simulink model "qpsk_rx_ssr_hb_decim"  (R2020a)
settings: Solver=VariableStepAuto  StartTime=0.0  StopTime=10000/64e6  RelTol=1e-3
PreLoadFcn:
  | setup_qpsk_receiver
InitFcn:
  | setup_qpsk_receiver
values from neighbouring files (symbols this model uses):
  tx_data = [tx_data mbuf]    [setup_receiver.m]
undefined symbols (not defined in the file or in its folder): designMultirateFIR, xlfda_numerator
libraries: xbsIndex_r4 x13, hdlsllib x9, dspmlti4 x8, xrbsSSR_Library x4, dspswit3 x4, commrandsrc3 x2, dspsigops x2, simulink x1
(part 1 of 2)
settings Model: Creator=david  LastModifiedBy=david
settings SFSimCC: CustomCodeUndefinedFunction=UseInterfaceOnly

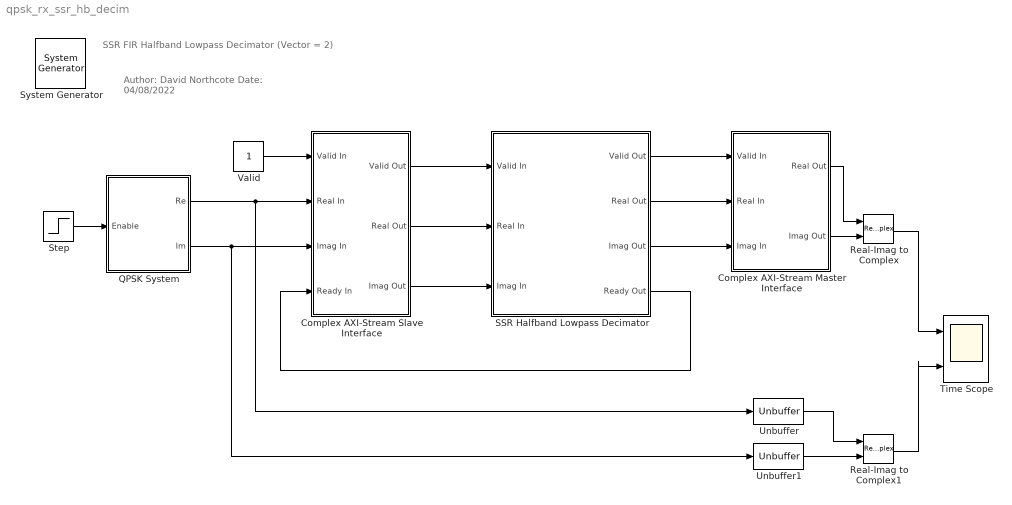
== system qpsk_rx_ssr_hb_decim ==
  note: Author: 	David Northcote
      | Date: 	04/08/2022
  note: SSR FIR Halfband Lowpass Decimator (Vector = 2)
  " System Generator" : xbsIndex_r4/ System Generator  Tag=genX  xilinxfamily=zynquplusRFSOC  part=xczu28dr  speed=-2-e  package=ffvg1517  synthesis_tool=Vivado  clock_wrapper=Clock Enables  directory=./netlist  proj_type=Vivado  Synth_file=Vivado Synthesis Defaults  Impl_file=Vivado Implementation Defaults  testbench=off  simulink_period=1/64e6  sysclk_period=(1/64e6)*1e9  dcm_input_clock_period=10  incr_netlist=off  trim_vbits=Everywhere in SubSystem  dbl_ovrd=According to Block Masks  core_generation=According to Block Masks  run_coregen=off  deprecated_control=off  eval_field=0  block_type=sysgen
  Complex AXI-Stream Master Interface : Subsystem
  Complex AXI-Stream Slave Interface : Subsystem
  QPSK System : Subsystem
  Real-Imag to Complex : RealImagToComplex
  Real-Imag to Complex1 : RealImagToComplex
  SSR Halfband Lowpass Decimator : Subsystem
  Step : Step  Time=2/25e3  SampleTime=1/25e3
  Time Scope : Scope  NumInputPorts=2
  Unbuffer : Unbuffer
  Unbuffer1 : Unbuffer
  Valid : Constant  OutDataTypeStr=boolean  SampleTime=1/64e6
  wires:
  QPSK System/1(Re) -> Unbuffer/1, Complex AXI-Stream Slave Interface/2(Real In)
  QPSK System/2(Im) -> Unbuffer1/1, Complex AXI-Stream Slave Interface/3(Imag In)
  Step/1 -> QPSK System/1(Enable)
  Unbuffer1/1 -> Real-Imag to Complex1/2
  Unbuffer/1 -> Real-Imag to Complex1/1
  Real-Imag to Complex1/1 -> Time Scope/2
  Real-Imag to Complex/1 -> Time Scope/1
  SSR Halfband Lowpass Decimator/1(Valid Out) -> Complex AXI-Stream Master Interface/1(Valid In)
  SSR Halfband Lowpass Decimator/2(Real Out) -> Complex AXI-Stream Master Interface/2(Real In)
  SSR Halfband Lowpass Decimator/3(Imag Out) -> Complex AXI-Stream Master Interface/3(Imag In)
  Complex AXI-Stream Master Interface/1(Real Out) -> Real-Imag to Complex/1
  Complex AXI-Stream Master Interface/2(Imag Out) -> Real-Imag to Complex/2
  Valid/1 -> Complex AXI-Stream Slave Interface/1(Valid In)
  SSR Halfband Lowpass Decimator/4(Ready Out) -> Complex AXI-Stream Slave Interface/4(Ready In)
  Complex AXI-Stream Slave Interface/1(Valid Out) -> SSR Halfband Lowpass Decimator/1(Valid In)
  Complex AXI-Stream Slave Interface/2(Real Out) -> SSR Halfband Lowpass Decimator/2(Real In)
  Complex AXI-Stream Slave Interface/3(Imag Out) -> SSR Halfband Lowpass Decimator/3(Imag In)

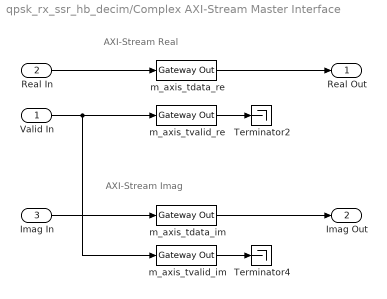
== system qpsk_rx_ssr_hb_decim/Complex AXI-Stream Master Interface ==
  note: AXI-Stream Real
  note: AXI-Stream Imag
  Valid In : Inport
  Real In : Inport  Port=2
  Imag In : Inport  Port=3
  Terminator2 : Terminator
  Terminator4 : Terminator
  m_axis_tdata_im : xbsIndex_r4/Gateway Out  inherit_from_input=off  hdl_port=on  rows=1  columns=1  UseAsDAC=off  DACChannel='1'  interface=None  automatic_assignment=on  address_offset=hex2dec('00')  intf_name=''  intf_description=''  timing_constraint=None  locs_specified=off  LOCs={}  io_standard={}  block_type=gatewayout
  m_axis_tdata_re : xbsIndex_r4/Gateway Out  inherit_from_input=off  hdl_port=on  rows=1  columns=1  UseAsDAC=off  DACChannel='1'  interface=None  automatic_assignment=on  address_offset=hex2dec('00')  intf_name=''  intf_description=''  timing_constraint=None  locs_specified=off  LOCs={}  io_standard={}  block_type=gatewayout
  m_axis_tvalid_im : xbsIndex_r4/Gateway Out  inherit_from_input=off  hdl_port=on  rows=1  columns=1  UseAsDAC=off  DACChannel='1'  interface=None  automatic_assignment=on  address_offset=hex2dec('00')  intf_name=''  intf_description=''  timing_constraint=None  locs_specified=off  LOCs={}  io_standard={}  block_type=gatewayout
  m_axis_tvalid_re : xbsIndex_r4/Gateway Out  inherit_from_input=off  hdl_port=on  rows=1  columns=1  UseAsDAC=off  DACChannel='1'  interface=None  automatic_assignment=on  address_offset=hex2dec('00')  intf_name=''  intf_description=''  timing_constraint=None  locs_specified=off  LOCs={}  io_standard={}  block_type=gatewayout
  Real Out : Outport  VectorParamsAs1DForOutWhenUnconnected=off
  Imag Out : Outport  Port=2  VectorParamsAs1DForOutWhenUnconnected=off
  wires:
  Real In/1 -> m_axis_tdata_re/1
  m_axis_tdata_im/1 -> Imag Out/1
  m_axis_tvalid_im/1 -> Terminator4/1
  Valid In/1 -> m_axis_tvalid_re/1, m_axis_tvalid_im/1
  m_axis_tdata_re/1 -> Real Out/1
  m_axis_tvalid_re/1 -> Terminator2/1
  Imag In/1 -> m_axis_tdata_im/1

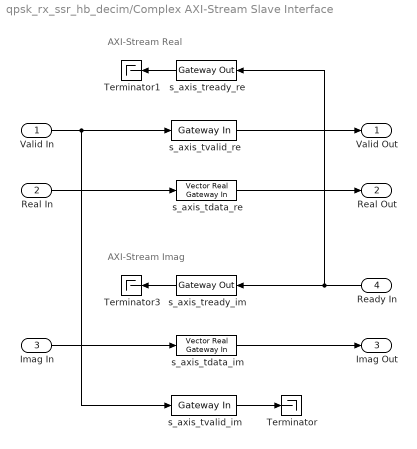
== system qpsk_rx_ssr_hb_decim/Complex AXI-Stream Slave Interface ==
  note: AXI-Stream Real
  note: AXI-Stream Imag
  Valid In : Inport
  Real In : Inport  Port=2
  Imag In : Inport  Port=3
  Ready In : Inport  Port=4
  Terminator : Terminator
  Terminator1 : Terminator
  Terminator3 : Terminator
  s_axis_tdata_im : xrbsSSR_Library/Vector Real Gateway In  gui_display_data_type=Fixed-point  arith_type="Signed  (2's comp)"  n_bits=16  bin_pt=14  preci_type=Single  exp_width=8  frac_width=24  quantization="Round  (unbiased: +/- Inf)"  overflow=Saturate  period=1/64e6  sg_ssr=2  sg_ssr_prev=2  UseAsADC=off  ADCChannel='1'  interface=None  interface_prev=1  automatic_assignment=off  address_offset=hex2dec('00')  intf_name=''  intf_description=''  default_value=0  timing_constraint=None  locs_specified=off  LOCs={}  io_standard={}  hdl_port=on  dbl_ovrd=off  block_type=realgatewayin_ssr
      settings: SourceProductName=Xilinx SSR Blockset  infoedit=The Vector Real Gateway in block converts Vector inputs of type Simulink integer, single, double and fixed-point to Xilinx fixed-point or floating-point data type.<br><br>Hardware notes: In hardware these blocks become top level input ports.
  s_axis_tdata_re : xrbsSSR_Library/Vector Real Gateway In  gui_display_data_type=Fixed-point  arith_type="Signed  (2's comp)"  n_bits=16  bin_pt=14  preci_type=Single  exp_width=8  frac_width=24  quantization="Round  (unbiased: +/- Inf)"  overflow=Saturate  period=1/64e6  sg_ssr=2  sg_ssr_prev=2  UseAsADC=off  ADCChannel='1'  interface=None  interface_prev=1  automatic_assignment=off  address_offset=hex2dec('00')  intf_name=''  intf_description=''  default_value=0  timing_constraint=None  locs_specified=off  LOCs={}  io_standard={}  hdl_port=on  dbl_ovrd=off  block_type=realgatewayin_ssr
      settings: SourceProductName=Xilinx SSR Blockset  infoedit=The Vector Real Gateway in block converts Vector inputs of type Simulink integer, single, double and fixed-point to Xilinx fixed-point or floating-point data type.<br><br>Hardware notes: In hardware these blocks become top level input ports.
  s_axis_tready_im : xbsIndex_r4/Gateway Out  inherit_from_input=off  hdl_port=on  rows=1  columns=1  UseAsDAC=off  DACChannel='1'  interface=None  automatic_assignment=on  address_offset=hex2dec('00')  intf_name=''  intf_description=''  timing_constraint=None  locs_specified=off  LOCs={}  io_standard={}  block_type=gatewayout
  s_axis_tready_re : xbsIndex_r4/Gateway Out  inherit_from_input=off  hdl_port=on  rows=1  columns=1  UseAsDAC=off  DACChannel='1'  interface=None  automatic_assignment=on  address_offset=hex2dec('00')  intf_name=''  intf_description=''  timing_constraint=None  locs_specified=off  LOCs={}  io_standard={}  block_type=gatewayout
  s_axis_tvalid_im : xbsIndex_r4/Gateway In  gui_display_data_type=Boolean  arith_type=Boolean  n_bits=16  bin_pt=14  preci_type=Single  exp_width=8  frac_width=24  rows=1  columns=1  quantization="Round  (unbiased: +/- Inf)"  overflow=Saturate  period=1/64e6  UseAsADC=off  ADCChannel='1'  interface=None  automatic_assignment=on  address_offset=hex2dec('00')  intf_name=''  intf_description=''  default_value=0  timing_constraint=None  locs_specified=off  LOCs={}  io_standard={}  inherit_from_input=off  hdl_port=on  dbl_ovrd=off  block_type=gatewayin
  s_axis_tvalid_re : xbsIndex_r4/Gateway In  gui_display_data_type=Boolean  arith_type=Boolean  n_bits=16  bin_pt=14  preci_type=Single  exp_width=8  frac_width=24  rows=1  columns=1  quantization="Round  (unbiased: +/- Inf)"  overflow=Saturate  period=1/64e6  UseAsADC=off  ADCChannel='1'  interface=None  automatic_assignment=on  address_offset=hex2dec('00')  intf_name=''  intf_description=''  default_value=0  timing_constraint=None  locs_specified=off  LOCs={}  io_standard={}  inherit_from_input=off  hdl_port=on  dbl_ovrd=off  block_type=gatewayin
  Valid Out : Outport  VectorParamsAs1DForOutWhenUnconnected=off
  Real Out : Outport  Port=2  VectorParamsAs1DForOutWhenUnconnected=off
  Imag Out : Outport  Port=3  VectorParamsAs1DForOutWhenUnconnected=off
  wires:
  Imag In/1 -> s_axis_tdata_im/1
  s_axis_tready_re/1 -> Terminator1/1
  s_axis_tdata_re/1 -> Real Out/1
  s_axis_tdata_im/1 -> Imag Out/1
  Valid In/1 -> s_axis_tvalid_re/1, s_axis_tvalid_im/1
  Ready In/1 -> s_axis_tready_im/1, s_axis_tready_re/1
  s_axis_tvalid_re/1 -> Valid Out/1
  s_axis_tvalid_im/1 -> Terminator/1
  s_axis_tready_im/1 -> Terminator3/1
  Real In/1 -> s_axis_tdata_re/1

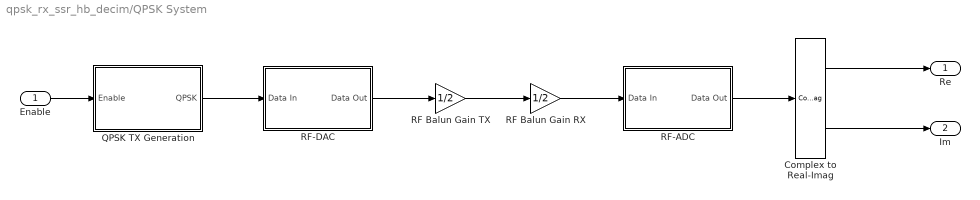
== system qpsk_rx_ssr_hb_decim/QPSK System ==
  Enable : Inport
  Complex to Real-Imag : ComplexToRealImag
  QPSK TX Generation : Subsystem
  RF Balun Gain RX : Gain  Gain=1/2
  RF Balun Gain TX : Gain  Gain=1/2
  RF-ADC : Subsystem  mask{fs_ghz=1.024, decim=8x, ssr=2, mode=Fine, fc=0.064, fph=0, fcoarse=fs/4}
      mask prompts: fs_ghz "Sample Rate (GHz):"; decim "Interpolation Mode:"; ssr "Samples per AXI4-Stream Cycle:"; mode "Mixer Type:"; fc "NCO Frequency (GHz):"; fph "NCO Phase (Rads):"; fcoarse "Frequency:"
      mask init:
      | % Obtain the sample rate in Hz
      | fs = str2double(get_param(gcb, 'fs_ghz'))*1e9;
      | 
      | % Set the mode of the RF-DAC interpolation filter
      | switch get_param(gcb, 'decim')
      |     case '1x'
      |         D = 1;
      |     case '2x'
      |         D = 2;
      |     case '4x'
      |         D = 4;
      |     case '8x'
      |         D = 8;
      |     otherwise
      |         D = 1;
      | end
      | 
      | % Get the AXI-Stream clock for display to user
      | axi_clk = (fs/(str2double(get_param(gcb, 'ssr'))*D))*1e-6;
      | 
      | % Get the block mask object to manipulate settings
      | mo = get_param(gcb, 'MaskObject');
      | 
      | % Update text to display the required AXI-Stream clock
      | tc = mo.getDialogControl('axi_text');
      | tc.Prompt = ['      Required AXI-Stream Clock: ', num2str(axi_clk), ' MHz'];
      | 
      | % Set the RF-DAC Mixer mode
      | switch get_param(gcb, 'mode')
      |     case 'Bypass'
      |         m = 0;
      |     case 'Coarse'
      |         m = 1;
      |     case 'Fine'
      |         m = 2;
      |     otherwise
      |         m = 0;
      | end
      | 
      | % Set the RF-DAC Coarse Mixer mode
      | switch get_param(gcb, 'fcoarse')
      |     case 'fs/2'
      |         mc = 0;
      |     case 'fs/4'
      |         mc = 1;
      |     case '-fs/4'
      |         mc = 2;
      |     otherwise
      |         mc = 0;
      | end
      | 
      | % Set other blocks
      | set_param([gcb, '/Decimation Filter'], 'decim', get_param(gcb, 'decim'));
      mask Callback fs_ghz:
      | % Obtain the sample rate in Hz
      | fs = str2double(get_param(gcb, 'fs_ghz'))*1e9;
      | 
      | % Set the mode of the RF-DAC interpolation filter
      | switch get_param(gcb, 'decim')
      |     case '1x'
      |         D = 1;
      |     case '2x'
      |         D = 2;
      |     case '4x'
      |         D = 4;
      |     case '8x'
      |         D = 8;
      |     otherwise
      |         D = 1;
      | end
      | 
      | % Get the AXI-Stream clock for display to user
      | axi_clk = (fs/(str2double(get_param(gcb, 'ssr'))*D))*1e-6;
      | 
      | % Get the block mask object to manipulate settings
      | mo = get_param(gcb, 'MaskObject');
      | 
      | % Update text to display the required AXI-Stream clock
      | tc = mo.getDialogControl('axi_text');
      | tc.Prompt = ['      Required AXI-Stream Clock: ', num2str(axi_clk), ' MHz'];
      mask TypeOptions decim: 1x | 2x | 4x | 8x
      mask Callback decim:
      | % Obtain the sample rate in Hz
      | fs = str2double(get_param(gcb, 'fs_ghz'))*1e9;
      | 
      | % Set the mode of the RF-DAC interpolation filter
      | switch get_param(gcb, 'decim')
      |     case '1x'
      |         D = 1;
      |     case '2x'
      |         D = 2;
      |     case '4x'
      |         D = 4;
      |     case '8x'
      |         D = 8;
      |     otherwise
      |         D = 1;
      | end
      | 
      | % Get the AXI-Stream clock for display to user
      | axi_clk = (fs/(str2double(get_param(gcb, 'ssr'))*D))*1e-6;
      | 
      | % Get the block mask object to manipulate settings
      | mo = get_param(gcb, 'MaskObject');
      | 
      | % Update text to display the required AXI-Stream clock
      | tc = mo.getDialogControl('axi_text');
      | tc.Prompt = ['      Required AXI-Stream Clock: ', num2str(axi_clk), ' MHz'];
      mask TypeOptions ssr: 1 | 2 | 3 | 4 | 5 | 6 | 7 | 8 | 9 | 10 | 11 | 12 | 13 | 14 | 15 | 16
      mask Callback ssr:
      | % Obtain the sample rate in Hz
      | fs = str2double(get_param(gcb, 'fs_ghz'))*1e9;
      | 
      | % Set the mode of the RF-DAC interpolation filter
      | switch get_param(gcb, 'decim')
      |     case '1x'
      |         D = 1;
      |     case '2x'
      |         D = 2;
      |     case '4x'
      |         D = 4;
      |     case '8x'
      |         D = 8;
      |     otherwise
      |         D = 1;
      | end
      | 
      | % Get the AXI-Stream clock for display to user
      | axi_clk = (fs/(str2double(get_param(gcb, 'ssr'))*D))*1e-6;
      | 
      | % Get the block mask object to manipulate settings
      | mo = get_param(gcb, 'MaskObject');
      | 
      | % Update text to display the required AXI-Stream clock
      | tc = mo.getDialogControl('axi_text');
      | tc.Prompt = ['      Required AXI-Stream Clock: ', num2str(axi_clk), ' MHz'];
      mask TypeOptions mode: Coarse | Fine
      mask Callback mode:
      | % Get the block mask object to manipulate settings
      | mo = get_param(gcb, 'MaskObject');
      | 
      | % Hide group depending on Mixer mode choice
      | switch get_param(gcb, 'mode')
      |     case 'Bypass'
      |         mo.getDialogControl('coarse_group').Visible='off';
      |         mo.getDialogControl('mixer_group').Visible='off';
      |     case 'Coarse'
      |         mo.getDialogControl('coarse_group').Visible='on';
      |         mo.getDialogControl('mixer_group').Visible='off';
      |     case 'Fine'
      |         mo.getDialogControl('coarse_group').Visible='off';
      |         mo.getDialogControl('mixer_group').Visible='on';
      |     otherwise
      |         mo.getDialogControl('coarse_group').Visible='off';
      |         mo.getDialogControl('mixer_group').Visible='off';
      | end
      mask TypeOptions fcoarse: fs/2 | fs/4 | -fs/4
      mask DialogControl DescGroupVar Prompt: RF-DAC
      mask DialogControl DescTextVar Prompt: This block simulates one RF-ADC channel.
      mask DialogControl main_group Prompt: Data Settings
      mask DialogControl axi_text Prompt: Required AXI-Stream Clock: 64 MHz
      mask DialogControl Container5 Prompt: Mixer Settings
  RF-DAC : Subsystem  mask{fs_ghz=1.024, interp=8x, ssr=1, mode=Fine, fc=0.064, fph=0, fcoarse=fs/4}
      mask prompts: fs_ghz "Sample Rate (GHz):"; interp "Interpolation Mode:"; ssr "Samples per AXI4-Stream Cycle:"; mode "Mixer Type:"; fc "NCO Frequency (GHz):"; fph "NCO Phase (Rads):"; fcoarse "Frequency:"
      mask init:
      | % Obtain the sample rate in Hz
      | fs = str2double(get_param(gcb, 'fs_ghz'))*1e9;
      | 
      | % Set the mode of the RF-DAC interpolation filter
      | switch get_param(gcb, 'interp')
      |     case '1x'
      |         L = 1;
      |     case '2x'
      |         L = 2;
      |     case '4x'
      |         L = 4;
      |     case '8x'
      |         L = 8;
      |     otherwise
      |         L = 1;
      | end
      | 
      | % Get the AXI-Stream clock for display to user
      | axi_clk = (fs/(str2double(get_param(gcb, 'ssr'))*L))*1e-6;
      | 
      | % Get the block mask object to manipulate settings
      | mo = get_param(gcb, 'MaskObject');
      | 
      | % Update text to display the required AXI-Stream clock
      | tc = mo.getDialogControl('axi_text');
      | tc.Prompt = ['      Required AXI-Stream Clock: ', num2str(axi_clk), ' MHz'];
      | 
      | % Set the RF-DAC Mixer mode
      | switch get_param(gcb, 'mode')
      |     case 'Bypass'
      |         m = 0;
      |     case 'Coarse'
      |         m = 1;
      |     case 'Fine'
      |         m = 2;
      |     otherwise
      |         m = 0;
      | end
      | 
      | % Set the RF-DAC Coarse Mixer mode
      | switch get_param(gcb, 'fcoarse')
      |     case 'fs/2'
      |         mc = 0;
      |     case 'fs/4'
      |         mc = 1;
      |     case '-fs/4'
      |         mc = 2;
      |     otherwise
      |         mc = 0;
      | end
      | 
      | % Set other blocks
      | set_param([gcb, '/Interpolation Filter'], 'interp', get_param(gcb, 'interp'));
      mask Callback fs_ghz:
      | % Obtain the sample rate in Hz
      | fs = str2double(get_param(gcb, 'fs_ghz'))*1e9;
      | 
      | % Set the mode of the RF-DAC interpolation filter
      | switch get_param(gcb, 'interp')
      |     case '1x'
      |         L = 1;
      |     case '2x'
      |         L = 2;
      |     case '4x'
      |         L = 4;
      |     case '8x'
      |         L = 8;
      |     otherwise
      |         L = 1;
      | end
      | 
      | % Get the AXI-Stream clock for display to user
      | axi_clk = (fs/(str2double(get_param(gcb, 'ssr'))*L))*1e-6;
      | 
      | % Get the block mask object to manipulate settings
      | mo = get_param(gcb, 'MaskObject');
      | 
      | % Update text to display the required AXI-Stream clock
      | tc = mo.getDialogControl('axi_text');
      | tc.Prompt = ['      Required AXI-Stream Clock: ', num2str(axi_clk), ' MHz'];
      mask TypeOptions interp: 1x | 2x | 4x | 8x
      mask Callback interp:
      | % Obtain the sample rate in Hz
      | fs = str2double(get_param(gcb, 'fs_ghz'))*1e9;
      | 
      | % Set the mode of the RF-DAC interpolation filter
      | switch get_param(gcb, 'interp')
      |     case '1x'
      |         L = 1;
      |     case '2x'
      |         L = 2;
      |     case '4x'
      |         L = 4;
      |     case '8x'
      |         L = 8;
      |     otherwise
      |         L = 1;
      | end
      | 
      | % Get the AXI-Stream clock for display to user
      | axi_clk = (fs/(str2double(get_param(gcb, 'ssr'))*L))*1e-6;
      | 
      | % Get the block mask object to manipulate settings
      | mo = get_param(gcb, 'MaskObject');
      | 
      | % Update text to display the required AXI-Stream clock
      | tc = mo.getDialogControl('axi_text');
      | tc.Prompt = ['      Required AXI-Stream Clock: ', num2str(axi_clk), ' MHz'];
      mask TypeOptions ssr: 1 | 2 | 3 | 4 | 5 | 6 | 7 | 8 | 9 | 10 | 11 | 12 | 13 | 14 | 15 | 16
      mask Callback ssr:
      | % Obtain the sample rate in Hz
      | fs = str2double(get_param(gcb, 'fs_ghz'))*1e9;
      | 
      | % Set the mode of the RF-DAC interpolation filter
      | switch get_param(gcb, 'interp')
      |     case '1x'
      |         L = 1;
      |     case '2x'
      |         L = 2;
      |     case '4x'
      |         L = 4;
      |     case '8x'
      |         L = 8;
      |     otherwise
      |         L = 1;
      | end
      | 
      | % Get the AXI-Stream clock for display to user
      | axi_clk = (fs/(str2double(get_param(gcb, 'ssr'))*L))*1e-6;
      | 
      | % Get the block mask object to manipulate settings
      | mo = get_param(gcb, 'MaskObject');
      | 
      | % Update text to display the required AXI-Stream clock
      | tc = mo.getDialogControl('axi_text');
      | tc.Prompt = ['      Required AXI-Stream Clock: ', num2str(axi_clk), ' MHz'];
      mask TypeOptions mode: Coarse | Fine
      mask Callback mode:
      | % Get the block mask object to manipulate settings
      | mo = get_param(gcb, 'MaskObject');
      | 
      | % Hide group depending on Mixer mode choice
      | switch get_param(gcb, 'mode')
      |     case 'Bypass'
      |         mo.getDialogControl('coarse_group').Visible='off';
      |         mo.getDialogControl('mixer_group').Visible='off';
      |     case 'Coarse'
      |         mo.getDialogControl('coarse_group').Visible='on';
      |         mo.getDialogControl('mixer_group').Visible='off';
      |     case 'Fine'
      |         mo.getDialogControl('coarse_group').Visible='off';
      |         mo.getDialogControl('mixer_group').Visible='on';
      |     otherwise
      |         mo.getDialogControl('coarse_group').Visible='off';
      |         mo.getDialogControl('mixer_group').Visible='off';
      | end
      mask TypeOptions fcoarse: fs/2 | fs/4 | -fs/4
      mask DialogControl DescGroupVar Prompt: RF-DAC
      mask DialogControl DescTextVar Prompt: This block simulates one RF-DAC channel.
      mask DialogControl main_group Prompt: Data Settings
      mask DialogControl axi_text Prompt: Required AXI-Stream Clock: 128 MHz
      mask DialogControl Container5 Prompt: Mixer Settings
  Re : Outport  VectorParamsAs1DForOutWhenUnconnected=off
  Im : Outport  Port=2  VectorParamsAs1DForOutWhenUnconnected=off
  wires:
  RF Balun Gain RX/1 -> RF-ADC/1(Data In)
  RF Balun Gain TX/1 -> RF Balun Gain RX/1
  RF-DAC/1(Data Out) -> RF Balun Gain TX/1
  RF-ADC/1(Data Out) -> Complex to Real-Imag/1
  Complex to Real-Imag/2 -> Im/1
  Complex to Real-Imag/1 -> Re/1
  Enable/1 -> QPSK TX Generation/1(Enable)
  QPSK TX Generation/1(QPSK) -> RF-DAC/1(Data In)

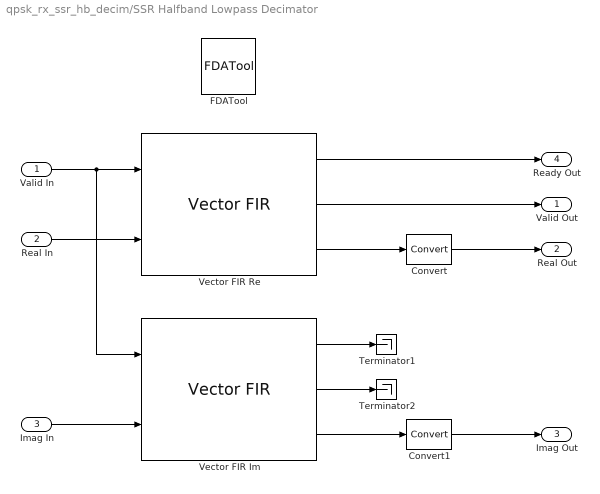
== system qpsk_rx_ssr_hb_decim/SSR Halfband Lowpass Decimator ==
  Valid In : Inport
  Real In : Inport  Port=2
  Imag In : Inport  Port=3
  Convert : xbsIndex_r4/Convert  gui_display_data_type=Fixed-point  arith_type="Signed  (2's comp)"  n_bits=16  bin_pt=14  float_type=Single  exp_bits=8  fraction_bits=24  quantization=Truncate  overflow=Wrap  en=off  latency=0  pipeline=off  dbl_ovrd=off  block_type=convert
  Convert1 : xbsIndex_r4/Convert  gui_display_data_type=Fixed-point  arith_type="Signed  (2's comp)"  n_bits=16  bin_pt=14  float_type=Single  exp_bits=8  fraction_bits=24  quantization=Truncate  overflow=Wrap  en=off  latency=0  pipeline=off  dbl_ovrd=off  block_type=convert
  FDATool : xbsIndex_r4/FDATool  block_type=fdatool
      settings: infoedit=FDATool
  Terminator1 : Terminator
  Terminator2 : Terminator
  Vector FIR Im : xrbsSSR_Library/Vector FIR  coefficientvector=xlfda_numerator('FDATool')/(max(xlfda_numerator('FDATool'))*2)  coefficient_sets=1  coeffsets_prev=1  coefficient_reload=off  filter_type=Decimation  filter_prev=Decimation  interpolation_rate=2  interpolation_prev=2  rate_change_type=Integer  decimation_rate=2  decimation_prev=2  zero_pack_factor=2  channel_sequence=Basic  number_channels=1  pattern_list='P4-0,P4-1,P4-2,P4-3,P4-4'  number_paths=1  sg_ssr=2  coefficient_sign=Signed  quantization=Quantize_Only  coefficient_width=16  bestprecision=off  coefficient_fractional_bits=14  coefficient_structure=Inferred  output_rounding_mode=Full_Precision  output_width=24  filter_architecture=Systolic_Multiply_Accumulate  optimization_goal=Area  optimization_list='None'  data_buffer_type=Automatic  coefficient_buffer_type=Automatic  input_buffer_type=Automatic  output_buffer_type=Automatic  preference_for_other_storage=Automatic  multi_column_support=Automatic  columnconfig='11'  inter_column_pipe_length=4  data_has_tlast=Not_Required  m_data_has_tready=off  s_data_has_fifo=off  s_data_has_tuser=Not_Required  m_data_has_tuser=Not_Required  s_config_sync_mode=On_Vector  s_config_method=Single  num_reload_slots=1  has_aclken=off  has_aresetn=off  infoeditControl=ARESETn must be asserted for a minimum of 2 cycles  reset_data_vector=on  simulation_type=xsim  simulation_model=sysgen:xfirv7_2_cmodel  data_path_portlist={ 's_axis_data_tdata', 'm_axis_data_tdata' }  passband_min=0.0  passband_max=0.5  stopband_min=0.5  stopband_max=1.0  filter_selection=1  gui_behaviour=1  data_sign=Signed  data_width=16  data_fractional_bits=0  data_tuser_width='11'  wrapper_available=true  ip_wrap_arbitrary_binary_point=true  ip_name=FIR Compiler  ip_version=7.2  dsptool_ready=true  ipcore_usecache=true  ipcore_useipmodelcache=true  port_translation_map={ 'aclken' => 'en', 'aresetn' => 'rst' }  run_core_at_system_period=true  ipcore_xco_need_fpga_part=true  ipcore_fpga_part=[]  block_type=fir_compiler_v7_2_ssr  sg_ssr_name=vect_FIR  sg_ssr_prev=2
      settings: SourceProductName=Xilinx SSR Blockset
  Vector FIR Re : xrbsSSR_Library/Vector FIR  coefficientvector=xlfda_numerator('FDATool')/(max(xlfda_numerator('FDATool'))*2)  coefficient_sets=1  coeffsets_prev=1  coefficient_reload=off  filter_type=Decimation  filter_prev=Decimation  interpolation_rate=2  interpolation_prev=2  rate_change_type=Integer  decimation_rate=2  decimation_prev=2  zero_pack_factor=2  channel_sequence=Basic  number_channels=1  pattern_list='P4-0,P4-1,P4-2,P4-3,P4-4'  number_paths=1  sg_ssr=2  coefficient_sign=Signed  quantization=Quantize_Only  coefficient_width=16  bestprecision=off  coefficient_fractional_bits=14  coefficient_structure=Inferred  output_rounding_mode=Full_Precision  output_width=24  filter_architecture=Systolic_Multiply_Accumulate  optimization_goal=Area  optimization_list='None'  data_buffer_type=Automatic  coefficient_buffer_type=Automatic  input_buffer_type=Automatic  output_buffer_type=Automatic  preference_for_other_storage=Automatic  multi_column_support=Automatic  columnconfig='11'  inter_column_pipe_length=4  data_has_tlast=Not_Required  m_data_has_tready=off  s_data_has_fifo=off  s_data_has_tuser=Not_Required  m_data_has_tuser=Not_Required  s_config_sync_mode=On_Vector  s_config_method=Single  num_reload_slots=1  has_aclken=off  has_aresetn=off  infoeditControl=ARESETn must be asserted for a minimum of 2 cycles  reset_data_vector=on  simulation_type=xsim  simulation_model=sysgen:xfirv7_2_cmodel  data_path_portlist={ 's_axis_data_tdata', 'm_axis_data_tdata' }  passband_min=0.0  passband_max=0.5  stopband_min=0.5  stopband_max=1.0  filter_selection=1  gui_behaviour=1  data_sign=Signed  data_width=16  data_fractional_bits=0  data_tuser_width='11'  wrapper_available=true  ip_wrap_arbitrary_binary_point=true  ip_name=FIR Compiler  ip_version=7.2  dsptool_ready=true  ipcore_usecache=true  ipcore_useipmodelcache=true  port_translation_map={ 'aclken' => 'en', 'aresetn' => 'rst' }  run_core_at_system_period=true  ipcore_xco_need_fpga_part=true  ipcore_fpga_part=[]  block_type=fir_compiler_v7_2_ssr  sg_ssr_name=vect_FIR  sg_ssr_prev=2
      settings: SourceProductName=Xilinx SSR Blockset
  Valid Out : Outport  VectorParamsAs1DForOutWhenUnconnected=off
  Real Out : Outport  Port=2  VectorParamsAs1DForOutWhenUnconnected=off
  Imag Out : Outport  Port=3  VectorParamsAs1DForOutWhenUnconnected=off
  Ready Out : Outport  Port=4  VectorParamsAs1DForOutWhenUnconnected=off
  wires:
  Imag In/1 -> Vector FIR Im/2
  Valid In/1 -> Vector FIR Im/1, Vector FIR Re/1
  Vector FIR Re/2 -> Valid Out/1
  Real In/1 -> Vector FIR Re/2
  Vector FIR Re/3 -> Convert/1
  Vector FIR Im/3 -> Convert1/1
  Vector FIR Im/1 -> Terminator1/1
  Vector FIR Re/1 -> Ready Out/1
  Vector FIR Im/2 -> Terminator2/1
  Convert/1 -> Real Out/1
  Convert1/1 -> Imag Out/1

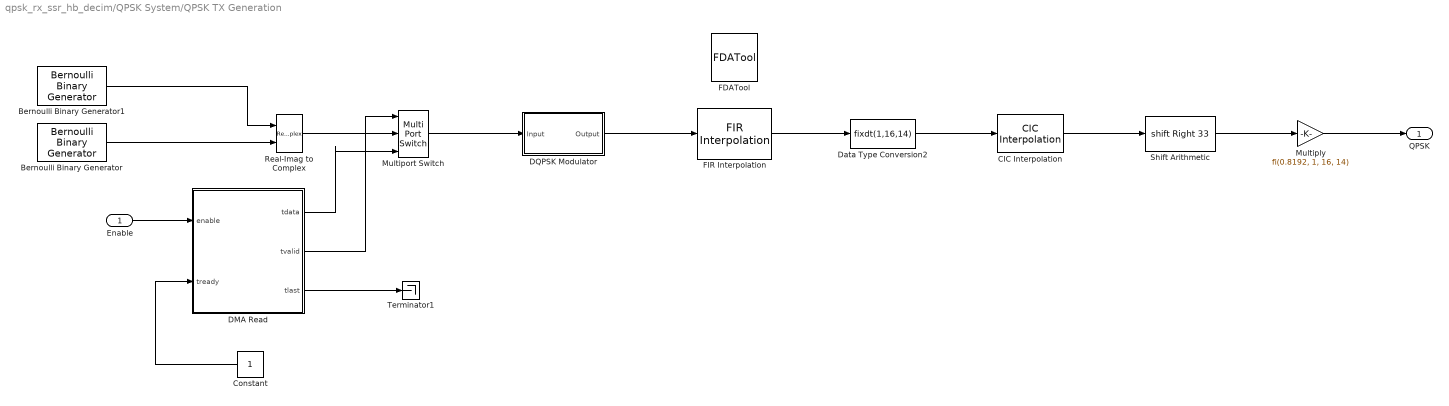
== system qpsk_rx_ssr_hb_decim/QPSK System/QPSK TX Generation ==
  Enable : Inport
  Bernoulli Binary Generator : commrandsrc3/Bernoulli Binary Generator  ProbabilityOfZero=0.5  SeedSource=Parameter  Seed=53  SampleTime=1/100e3  SamplesPerFrame=1  OutputDataType=double  SimulateUsing=Interpreted execution
  Bernoulli Binary Generator1 : commrandsrc3/Bernoulli Binary Generator  ProbabilityOfZero=0.5  SeedSource=Parameter  Seed=1  SampleTime=1/100e3  SamplesPerFrame=1  OutputDataType=double  SimulateUsing=Interpreted execution
  CIC Interpolation : dspmlti4/CIC Interpolation  filtFrom=Dialog parameters  filtobj=Hm_interp  ftype=Interpolator  R=320  M=1  N=5  filterInternals=Full precision  BPS=[16 16 16 16]  FLPS=0  outputWordLength=32  outputFracLength=0  launchFVT=off  framing=Allow multirate processing  OutputFrames=off
      settings: SourceProductBaseCode=DS
  Constant : Constant  SampleTime=1/25e3
  DMA Read : Subsystem
  DQPSK Modulator : Subsystem
  Data Type Conversion2 : DataTypeConversion  OutDataTypeStr=fixdt(1,16,14)
  FDATool : xbsIndex_r4/FDATool  block_type=fdatool
      settings: infoedit=FDATool
  FIR Interpolation : dspmlti4/FIR Interpolation  FilterSource=Dialog parameters  PrivateCoeffs=0  h=xlfda_numerator('FDATool')*4  L=4  FilterObject=xlfda_numerator('FDATool')/(max(xlfda_numerator('FDATool')))  framing=Allow multirate processing  outputBufInitCond=0  roundingMode=Floor  overflowMode=off  firstCoeffMode=Binary point scaling  firstCoeffWordLength=16  firstCoeffFracLength=14  firstCoeffDataTypeStr=fixdt(1,16,14)  firstCoeffMin=[]  firstCoeffMax=[]  firstCoeffLastDataTypeStr=fixdt(1,16,14)  outputDataTypeStr=Inherit: Same as accumulator  outputMin=[]  outputMax=[]  outputLastDataTypeStr=Inherit: Same as accumulator
  Multiply : Gain  Gain=fi(0.8192, 1, 16, 14)  ParamDataTypeStr=fixdt(1,16,15)  OutDataTypeStr=fixdt(1,16,14)
  Multiport Switch : MultiPortSwitch  DataPortOrder=Zero-based contiguous  Inputs=2  zeroidx=on
  Real-Imag to Complex : RealImagToComplex
  Shift Arithmetic : ArithShift  BitShiftNumber=33  BitShiftDirection=Right
  Terminator1 : Terminator
  QPSK : Outport  VectorParamsAs1DForOutWhenUnconnected=off
  wires:
  Shift Arithmetic/1 -> Multiply/1
  Data Type Conversion2/1 -> CIC Interpolation/1
  DQPSK Modulator/1(Output) -> FIR Interpolation/1
  Multiply/1 -> QPSK/1
  Multiport Switch/1 -> DQPSK Modulator/1(Input)
  Constant/1 -> DMA Read/2(tready)
  Enable/1 -> DMA Read/1(enable)
  DMA Read/3(tlast) -> Terminator1/1
  DMA Read/1(tdata) -> Multiport Switch/3
  DMA Read/2(tvalid) -> Multiport Switch/1
  FIR Interpolation/1 -> Data Type Conversion2/1
  CIC Interpolation/1 -> Shift Arithmetic/1
  Bernoulli Binary Generator1/1 -> Real-Imag to Complex/1
  Bernoulli Binary Generator/1 -> Real-Imag to Complex/2
  Real-Imag to Complex/1 -> Multiport Switch/2

== system qpsk_rx_ssr_hb_decim/QPSK System/RF-ADC ==
  Data In : Inport
  Decimation Filter : Subsystem  mask{decim=8x}
      mask prompts: decim "Decimation Factor:"
      mask init:
      | fir0 = dsp.FIRDecimator('DecimationFactor', 2,...
      |                            'CoefficientsDataType', 'Custom',...
      |                            'CustomCoefficientsDataType', numerictype([], 16, 14),...
      |                            'FullPrecisionOverride', false,...
      |                            'OutputDataType', 'Custom',...
      |                            'CustomOutputDataType', numerictype([], 16, 14),...
      |                            'Numerator', [-6, 0 54, 0, -254, 0, 1230, 2048, 1230, 0, -254, 0, 54, 0, -6]/(2048*2));
      | fir1 = dsp.FIRDecimator('DecimationFactor', 2,...
      |                            'CoefficientsDataType', 'Custom',...
      |                            'CustomCoefficientsDataType', numerictype([], 16, 14),...
      |                            'FullPrecisionOverride', false,...
      |                            'OutputDataType', 'Custom',...
      |                            'CustomOutputDataType', numerictype([], 16, 14),...
      |                            'Numerator', [-12, 0, 84, 0, -337, 0, 1008, 0, -2693, 0, 10142, 16384, 10142, 0, -2693, 0, 1008, 0, -337, 0, 84, 0 ,-12]/(16384*2));
      | fir2 = dsp.FIRDecimator('DecimationFactor', 2,...
      |                            'CoefficientsDataType', 'Custom',...
      |                            'CustomCoefficientsDataType', numerictype([], 16, 14),...
      |                            'FullPrecisionOverride', false,...
      |                            'OutputDataType', 'Custom',...
      |                            'CustomOutputDataType', numerictype([], 16, 14),...
      |                            'Numerator', [5, 0, -17, 0, 44, 0, -96, 0, 187, 0, -335, 0, 565, 0, -906, 0, 1401, 0, -2112, 0, 3145, 0, -4723, 0, 7415, 0, -13331, 0, 41526, 65536, 41526, 0, -13331, 0, 7415, 0, -4723, 0, 3145, 0, -2112, 0, 1401, 0, -906, 0, 565, 0, -335, 0, 187, 0, -96, 0, 44, 0, -17, 0, 5]/(65536));
      | switch get_param(gcb, 'decim')
      |     case '1x'
      |         if ~strcmp(get_param([gcb, '/FIR 0'], 'Commented'), 'through')
      |             set_param([gcb, '/FIR 0'],'Commented','through');
      |         end
      |         
      |         if ~strcmp(get_param([gcb, '/FIR 1'], 'Commented'), 'through')
      |             set_param([gcb, '/FIR 1'],'Commented','through');
      |         end
      |         
      |         if ~strcmp(get_param([gcb, '/FIR 2'], 'Commented'), 'through')
      |             set_param([gcb, '/FIR 2'],'Commented','through');
      |         end
      |             
      |     case '2x'
      |         if ~strcmp(get_param([gcb, '/FIR 0'], 'Commented'), 'through')
      |             set_param([gcb, '/FIR 0'],'Commented','through');
      |         end
      |         
      |         if ~strcmp(get_param([gcb, '/FIR 1'], 'Commented'), 'through')
      |             set_param([gcb, '/FIR 1'],'Commented','through');
      |         end
      |         
      |         if ~strcmp(get_param([gcb, '/FIR 2'], 'Commented'), 'off')
      |             set_param([gcb, '/FIR 2'],'Commented','off');
      |         end
      | 
      |     case '4x'
      |         if ~strcmp(get_param([gcb, '/FIR 0'], 'Commented'), 'through')
      |             set_param([gcb, '/FIR 0'],'Commented','through');
      |         end
      |         
      |         if ~strcmp(get_param([gcb, '/FIR 1'], 'Commented'), 'off')
      |             set_param([gcb, '/FIR 1'],'Commented','off');
      |         end
      |         
      |         if ~strcmp(get_param([gcb, '/FIR 2'], 'Commented'), 'off')
      |             set_param([gcb, '/FIR 2'],'Commented','off');
      |         end
      |         
      |     case '8x'
      |         if ~strcmp(get_param([gcb, '/FIR 0'], 'Commented'), 'off')
      |             set_param([gcb, '/FIR 0'],'Commented','off');
      |         end
      |         
      |         if ~strcmp(get_param([gcb, '/FIR 1'], 'Commented'), 'off')
      |             set_param([gcb, '/FIR 1'],'Commented','off');
      |         end
      |         
      |         if ~strcmp(get_param([gcb, '/FIR 2'], 'Commented'), 'off')
      |             set_param([gcb, '/FIR 2'],'Commented','off');
      |         end
      | 
      | end
      mask TypeOptions decim: 1x | 2x | 4x | 8x
      mask DialogControl DescGroupVar Prompt: RF-DAC Interpolation Filter
      mask DialogControl DescTextVar Prompt: This block simulates the RF-DAC interpolation stage using the same coefficients stored in the interpolation filters.
      mask DialogControl ParameterGroupVar Prompt: Main
  NCO and Mixer : Subsystem
  RF-ADC : Subsystem
  Data Out : Outport  VectorParamsAs1DForOutWhenUnconnected=off
  wires:
  Decimation Filter/1(Data Out) -> Data Out/1
  Data In/1 -> RF-ADC/1(Data In)
  RF-ADC/1(Data Out) -> NCO and Mixer/1(Data In)
  NCO and Mixer/1(Data Out) -> Decimation Filter/1(Data In)

== system qpsk_rx_ssr_hb_decim/QPSK System/RF-DAC ==
  note: Not Ready
  Data In : Inport
  Coarse Delay : Subsystem
  Interpolation Filter : Subsystem  mask{interp=8x}
      mask prompts: interp "Interpolation Factor:"
      mask init:
      | fir0 = dsp.FIRInterpolator('InterpolationFactor', 2,...
      |                            'CoefficientsDataType', 'Custom',...
      |                            'CustomCoefficientsDataType', numerictype([], 16, 14),...
      |                            'FullPrecisionOverride', false,...
      |                            'OutputDataType', 'Custom',...
      |                            'CustomOutputDataType', numerictype([], 16, 14),...
      |                            'Numerator', [-6, 0 54, 0, -254, 0, 1230, 2048, 1230, 0, -254, 0, 54, 0, -6]/(2048));
      | fir1 = dsp.FIRInterpolator('InterpolationFactor', 2,...
      |                            'CoefficientsDataType', 'Custom',...
      |                            'CustomCoefficientsDataType', numerictype([], 16, 14),...
      |                            'FullPrecisionOverride', false,...
      |                            'OutputDataType', 'Custom',...
      |                            'CustomOutputDataType', numerictype([], 16, 14),...
      |                            'Numerator', [-12, 0, 84, 0, -337, 0, 1008, 0, -2693, 0, 10142, 16384, 10142, 0, -2693, 0, 1008, 0, -337, 0, 84, 0 ,-12]/(16384));
      | fir2 = dsp.FIRInterpolator('InterpolationFactor', 2,...
      |                            'CoefficientsDataType', 'Custom',...
      |                            'CustomCoefficientsDataType', numerictype([], 16, 14),...
      |                            'FullPrecisionOverride', false,...
      |                            'OutputDataType', 'Custom',...
      |                            'CustomOutputDataType', numerictype([], 16, 14),...
      |                            'Numerator', [5, 0, -17, 0, 44, 0, -96, 0, 187, 0, -335, 0, 565, 0, -906, 0, 1401, 0, -2112, 0, 3145, 0, -4723, 0, 7415, 0, -13331, 0, 41526, 65536, 41526, 0, -13331, 0, 7415, 0, -4723, 0, 3145, 0, -2112, 0, 1401, 0, -906, 0, 565, 0, -335, 0, 187, 0, -96, 0, 44, 0, -17, 0, 5]/(65536));
      | switch get_param(gcb, 'interp')
      |     case '1x'
      |         if ~strcmp(get_param([gcb, '/FIR 0'], 'Commented'), 'through')
      |             set_param([gcb, '/FIR 0'],'Commented','through');
      |         end
      |         
      |         if ~strcmp(get_param([gcb, '/FIR 1'], 'Commented'), 'through')
      |             set_param([gcb, '/FIR 1'],'Commented','through');
      |         end
      |         
      |         if ~strcmp(get_param([gcb, '/FIR 2'], 'Commented'), 'through')
      |             set_param([gcb, '/FIR 2'],'Commented','through');
      |         end
      |             
      |     case '2x'
      |         if ~strcmp(get_param([gcb, '/FIR 0'], 'Commented'), 'through')
      |             set_param([gcb, '/FIR 0'],'Commented','through');
      |         end
      |         
      |         if ~strcmp(get_param([gcb, '/FIR 1'], 'Commented'), 'through')
      |             set_param([gcb, '/FIR 1'],'Commented','through');
      |         end
      |         
      |         if ~strcmp(get_param([gcb, '/FIR 2'], 'Commented'), 'off')
      |             set_param([gcb, '/FIR 2'],'Commented','off');
      |         end
      | 
      |     case '4x'
      |         if ~strcmp(get_param([gcb, '/FIR 0'], 'Commented'), 'through')
      |             set_param([gcb, '/FIR 0'],'Commented','through');
      |         end
      |         
      |         if ~strcmp(get_param([gcb, '/FIR 1'], 'Commented'), 'off')
      |             set_param([gcb, '/FIR 1'],'Commented','off');
      |         end
      |         
      |         if ~strcmp(get_param([gcb, '/FIR 2'], 'Commented'), 'off')
      |             set_param([gcb, '/FIR 2'],'Commented','off');
      |         end
      |         
      |     case '8x'
      |         if ~strcmp(get_param([gcb, '/FIR 0'], 'Commented'), 'off')
      |             set_param([gcb, '/FIR 0'],'Commented','off');
      |         end
      |         
      |         if ~strcmp(get_param([gcb, '/FIR 1'], 'Commented'), 'off')
      |             set_param([gcb, '/FIR 1'],'Commented','off');
      |         end
      |         
      |         if ~strcmp(get_param([gcb, '/FIR 2'], 'Commented'), 'off')
      |             set_param([gcb, '/FIR 2'],'Commented','off');
      |         end
      | 
      | end
      mask TypeOptions interp: 1x | 2x | 4x | 8x
      mask DialogControl DescGroupVar Prompt: RF-DAC Interpolation Filter
      mask DialogControl DescTextVar Prompt: This block simulates the RF-DAC interpolation stage using the same coefficients stored in the interpolation filters.
      mask DialogControl ParameterGroupVar Prompt: Main
  NCO and Mixer : Subsystem
  Output Filter : Subsystem
  QMC Gain & Phase : Subsystem
  QMC Threshold : Subsystem
  RF-DAC : Subsystem
  Data Out : Outport  VectorParamsAs1DForOutWhenUnconnected=off
  wires:
  Interpolation Filter/1(Data Out) -> NCO and Mixer/1(Data In)
  NCO and Mixer/1(Data Out) -> QMC Gain & Phase/1(Data In)
  Data In/1 -> Interpolation Filter/1(Data In)
  QMC Gain & Phase/1(Data Out) -> Coarse Delay/1(Data In)
  Coarse Delay/1(Data Out) -> Output Filter/1(Data In)
  Output Filter/1(Data Out) -> QMC Threshold/1(Data In)
  QMC Threshold/1(Data Out) -> RF-DAC/1(Data In)
  RF-DAC/1(Data Out) -> Data Out/1

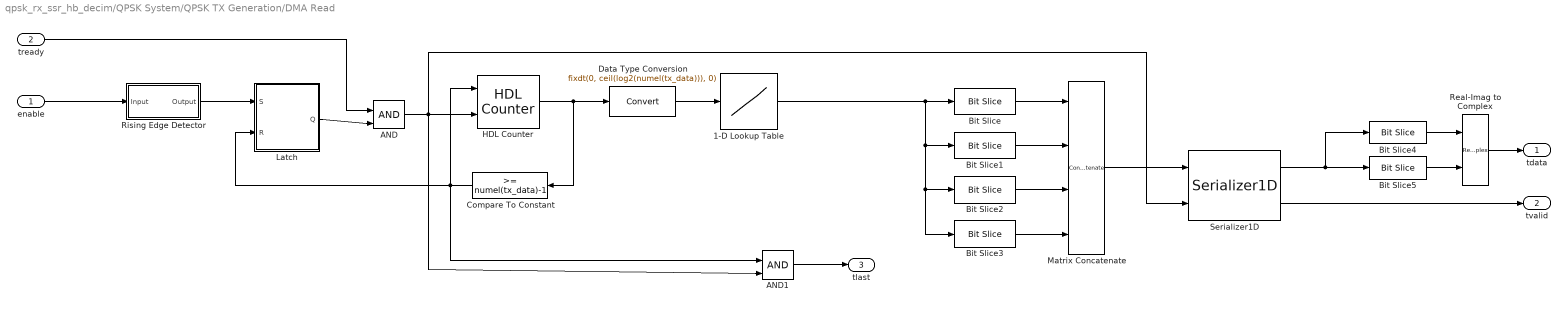
== system qpsk_rx_ssr_hb_decim/QPSK System/QPSK TX Generation/DMA Read ==
  enable : Inport
  tready : Inport  Port=2
  1-D Lookup Table : Lookup_n-D  NumberOfTableDimensions=1  BreakpointsForDimension1=[0:1:numel(tx_data)-1]  Table=tx_data  TableDataTypeStr=Inherit: Inherit from 'Table data'  ExtrapMethod=Clip  InternalRulePriority=Speed  OutDataTypeStr=Inherit: Inherit from 'Table data'  RndMeth=Simplest  InputSameDT=on
  AND : Logic  IconShape=distinctive  AllPortsSameDT=off  OutDataTypeStr=boolean
  AND1 : Logic  IconShape=distinctive  AllPortsSameDT=off  OutDataTypeStr=boolean
  Bit Slice : hdlsllib/Logic and Bit Operations/Bit Slice  lidx=1  ridx=0
      settings: SourceProductBaseCode=SL
  Bit Slice1 : hdlsllib/Logic and Bit Operations/Bit Slice  lidx=3  ridx=2
      settings: SourceProductBaseCode=SL
  Bit Slice2 : hdlsllib/Logic and Bit Operations/Bit Slice  lidx=5  ridx=4
      settings: SourceProductBaseCode=SL
  Bit Slice3 : hdlsllib/Logic and Bit Operations/Bit Slice  lidx=7  ridx=6
      settings: SourceProductBaseCode=SL
  Bit Slice4 : hdlsllib/Logic and Bit Operations/Bit Slice  lidx=0  ridx=0
      settings: SourceProductBaseCode=SL
  Bit Slice5 : hdlsllib/Logic and Bit Operations/Bit Slice  lidx=1  ridx=1
      settings: SourceProductBaseCode=SL
  Compare To Constant : simulink/Logic and Bit Operations/Compare To Constant  relop=>=  const=numel(tx_data)-1  OutDataTypeStr=boolean
  Data Type Conversion : DataTypeConversion  OutDataTypeStr=fixdt(0, ceil(log2(numel(tx_data))), 0)
  HDL Counter : hdlsllib/Sources/HDL Counter  CountType=Free running  CountInit=0  CountStep=1  CountMax=25  CountFromType=Initial value  CountFrom=0  CountResetPort=on  CountLoadPort=off  CountEnbPort=on  CountDirPort=off  CountDataType=Unsigned  CountWordLen=32  CountFracLen=0  CountSampTime=1
  Latch : Subsystem
  Matrix Concatenate : Concatenate  NumInputs=4  Mode=Multidimensional array  ConcatenateDimension=2
  Real-Imag to Complex : RealImagToComplex
  Rising Edge Detector : Subsystem
  Serializer1D : hdlsllib/HDL Operations/Serializer1D  Ratio=4  IdleCycles=0  validIn=on  startOut=off  validOut=on  inputDataDimensions=-1  inputSampleTime=-1  inputSignalType=auto
      settings: SourceProductBaseCode=SL
  tdata : Outport  VectorParamsAs1DForOutWhenUnconnected=off
  tvalid : Outport  Port=2  VectorParamsAs1DForOutWhenUnconnected=off
  tlast : Outport  Port=3  VectorParamsAs1DForOutWhenUnconnected=off
  wires:
  Serializer1D/2 -> tvalid/1
  1-D Lookup Table/1 -> Bit Slice/1, Bit Slice1/1, Bit Slice2/1, Bit Slice3/1
  Bit Slice2/1 -> Matrix Concatenate/3
  Bit Slice1/1 -> Matrix Concatenate/2
  Bit Slice3/1 -> Matrix Concatenate/4
  Bit Slice/1 -> Matrix Concatenate/1
  Matrix Concatenate/1 -> Serializer1D/1
  Compare To Constant/1 -> AND1/1, HDL Counter/1, Latch/2(R)
  enable/1 -> Rising Edge Detector/1(Input)
  HDL Counter/1 -> Compare To Constant/1, Data Type Conversion/1
  Data Type Conversion/1 -> 1-D Lookup Table/1
  Rising Edge Detector/1(Output) -> Latch/1(S)
  AND/1 -> AND1/2, Serializer1D/2, HDL Counter/2
  Latch/1(Q) -> AND/2
  tready/1 -> AND/1
  AND1/1 -> tlast/1
  Bit Slice4/1 -> Real-Imag to Complex/1
  Bit Slice5/1 -> Real-Imag to Complex/2
  Real-Imag to Complex/1 -> tdata/1
  Serializer1D/1 -> Bit Slice5/1, Bit Slice4/1

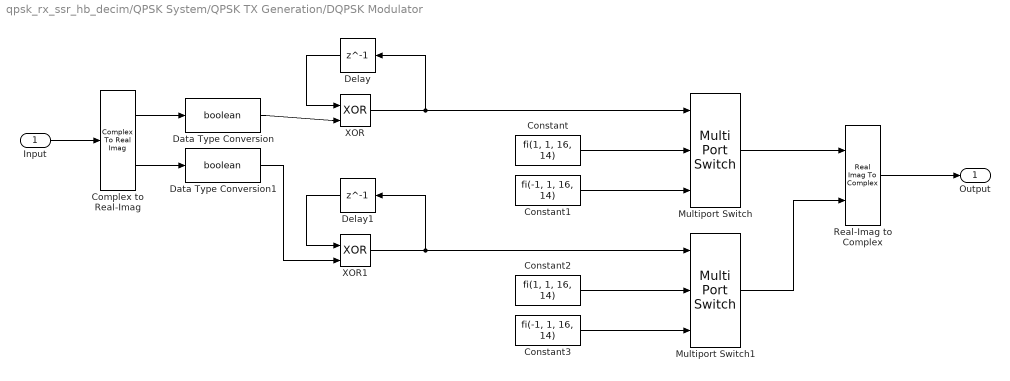
== system qpsk_rx_ssr_hb_decim/QPSK System/QPSK TX Generation/DQPSK Modulator ==
  Input : Inport
  Complex to Real-Imag : ComplexToRealImag
  Constant : Constant  Value=fi(1, 1, 16, 14)  OutDataTypeStr=fixdt(1,16,14)  SampleTime=-1
  Constant1 : Constant  Value=fi(-1, 1, 16, 14)  OutDataTypeStr=fixdt(1,16,14)  SampleTime=-1
  Constant2 : Constant  Value=fi(1, 1, 16, 14)  OutDataTypeStr=fixdt(1,16,14)  SampleTime=-1
  Constant3 : Constant  Value=fi(-1, 1, 16, 14)  OutDataTypeStr=fixdt(1,16,14)  SampleTime=-1
  Data Type Conversion : DataTypeConversion  OutDataTypeStr=boolean  RndMeth=Round
  Data Type Conversion1 : DataTypeConversion  OutDataTypeStr=boolean  RndMeth=Round
  Delay : Delay  DelayLength=1
  Delay1 : Delay  DelayLength=1
  Multiport Switch : MultiPortSwitch  DataPortOrder=Zero-based contiguous  Inputs=2  zeroidx=on
  Multiport Switch1 : MultiPortSwitch  DataPortOrder=Zero-based contiguous  Inputs=2  zeroidx=on
  Real-Imag to Complex : RealImagToComplex
  XOR : Logic  Operator=XOR  IconShape=distinctive  AllPortsSameDT=off  OutDataTypeStr=boolean
  XOR1 : Logic  Operator=XOR  IconShape=distinctive  AllPortsSameDT=off  OutDataTypeStr=boolean
  Output : Outport  VectorParamsAs1DForOutWhenUnconnected=off
  wires:
  Real-Imag to Complex/1 -> Output/1
  Multiport Switch/1 -> Real-Imag to Complex/1
  Constant1/1 -> Multiport Switch/3
  Constant/1 -> Multiport Switch/2
  Delay/1 -> XOR/1
  XOR/1 -> Multiport Switch/1, Delay/1
  Complex to Real-Imag/1 -> Data Type Conversion/1
  Input/1 -> Complex to Real-Imag/1
  Complex to Real-Imag/2 -> Data Type Conversion1/1
  XOR1/1 -> Delay1/1, Multiport Switch1/1
  Delay1/1 -> XOR1/1
  Constant2/1 -> Multiport Switch1/2
  Constant3/1 -> Multiport Switch1/3
  Multiport Switch1/1 -> Real-Imag to Complex/2
  Data Type Conversion/1 -> XOR/2
  Data Type Conversion1/1 -> XOR1/2

== system qpsk_rx_ssr_hb_decim/QPSK System/RF-ADC/Decimation Filter ==
  Data In : Inport
  FIR 0 : dspmlti4/FIR Decimation  FilterSource=Filter object  h=designMultirateFIR(1,2)  D=2  filtStruct=Direct form  FilterObject=fir0  InputProcessing=Columns as channels (frame based)  framing=Allow multirate processing  inputOffset=0  outputBufInitCond=0  roundingMode=Floor  overflowMode=off  firstCoeffDataTypeStr=Inherit: Same word length as input  firstCoeffMin=[]  firstCoeffMax=[]  firstCoeffLastDataTypeStr=Inherit: Same word length as input  outputDataTypeStr=Inherit: Same as accumulator  outputMin=[]  outputMax=[]  outputLastDataTypeStr=Inherit: Same as accumulator
  FIR 1 : dspmlti4/FIR Decimation  FilterSource=Filter object  h=designMultirateFIR(1,2)  D=2  filtStruct=Direct form  FilterObject=fir1  InputProcessing=Columns as channels (frame based)  framing=Allow multirate processing  inputOffset=0  outputBufInitCond=0  roundingMode=Floor  overflowMode=off  firstCoeffDataTypeStr=Inherit: Same word length as input  firstCoeffMin=[]  firstCoeffMax=[]  firstCoeffLastDataTypeStr=Inherit: Same word length as input  outputDataTypeStr=Inherit: Same as accumulator  outputMin=[]  outputMax=[]  outputLastDataTypeStr=Inherit: Same as accumulator
  FIR 2 : dspmlti4/FIR Decimation  FilterSource=Filter object  h=designMultirateFIR(1,2)  D=2  filtStruct=Direct form  FilterObject=fir2  InputProcessing=Columns as channels (frame based)  framing=Allow multirate processing  inputOffset=0  outputBufInitCond=0  roundingMode=Floor  overflowMode=off  firstCoeffDataTypeStr=Inherit: Same word length as input  firstCoeffMin=[]  firstCoeffMax=[]  firstCoeffLastDataTypeStr=Inherit: Same word length as input  outputDataTypeStr=Inherit: Same as accumulator  outputMin=[]  outputMax=[]  outputLastDataTypeStr=Inherit: Same as accumulator
  Data Out : Outport  VectorParamsAs1DForOutWhenUnconnected=off
  wires:
  FIR 2/1 -> FIR 1/1
  Data In/1 -> FIR 2/1
  FIR 0/1 -> Data Out/1
  FIR 1/1 -> FIR 0/1

== system qpsk_rx_ssr_hb_decim/QPSK System/RF-ADC/NCO and Mixer ==
  Data In : Inport
  Constant1 : Constant  Value=m  OutDataTypeStr=fixdt(0,2,0)  SampleTime=-1
  Data Type Conversion : DataTypeConversion  OutDataTypeStr=fixdt(1,16,14)
  Multiport Switch1 : MultiPortSwitch  DataPortOrder=Zero-based contiguous  zeroidx=on
  RF-ADC Coarse Mixer : Subsystem
  RF-ADC Fine Mixer : Subsystem
  Real-Imag to Complex : RealImagToComplex
  Data Out : Outport  VectorParamsAs1DForOutWhenUnconnected=off
  wires:
  Data Type Conversion/1 -> Multiport Switch1/2
  Constant1/1 -> Multiport Switch1/1
  Data In/1 -> Real-Imag to Complex/2, RF-ADC Fine Mixer/1(Data In), RF-ADC Coarse Mixer/1(Data In), Real-Imag to Complex/1
  RF-ADC Coarse Mixer/1(Data Out) -> Multiport Switch1/3
  Real-Imag to Complex/1 -> Data Type Conversion/1
  RF-ADC Fine Mixer/1(Data Out) -> Multiport Switch1/4
  Multiport Switch1/1 -> Data Out/1
